simulink subsystem "FTireTiresFront"  (R2025b)
settings: Solver=VariableStepAuto  StartTime=0.0  StopTime=10.0  RelTol=1e-3
undefined symbols (not defined in the file): PlntWhlPrsFrnt, PlntWhlUnldRadiusFrnt
libraries: ftire_link x2, autolibsharedcoupling x1, autolibutils x1, vehdynlibtirecommon x1
settings Model: ModifiedByFormat=The MathWorks, Inc.  Creator=The MathWorks, Inc.  LastModifiedBy=The MathWorks, Inc.
settings OptimizationCC: ReuseModelBlockBuffer=off
settings RTWCC: GPUComputeCapability=3.5

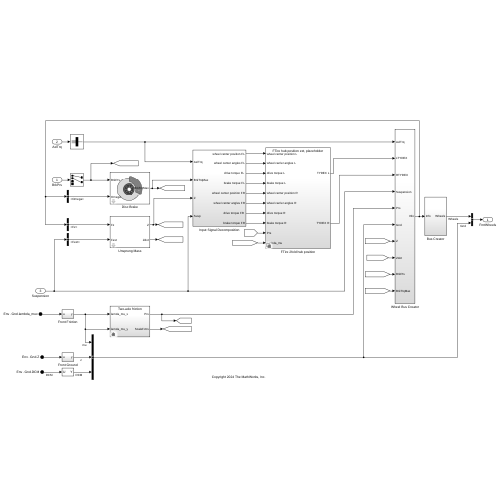
[thumbnail: Simulink's stored preview of the top-level diagram]
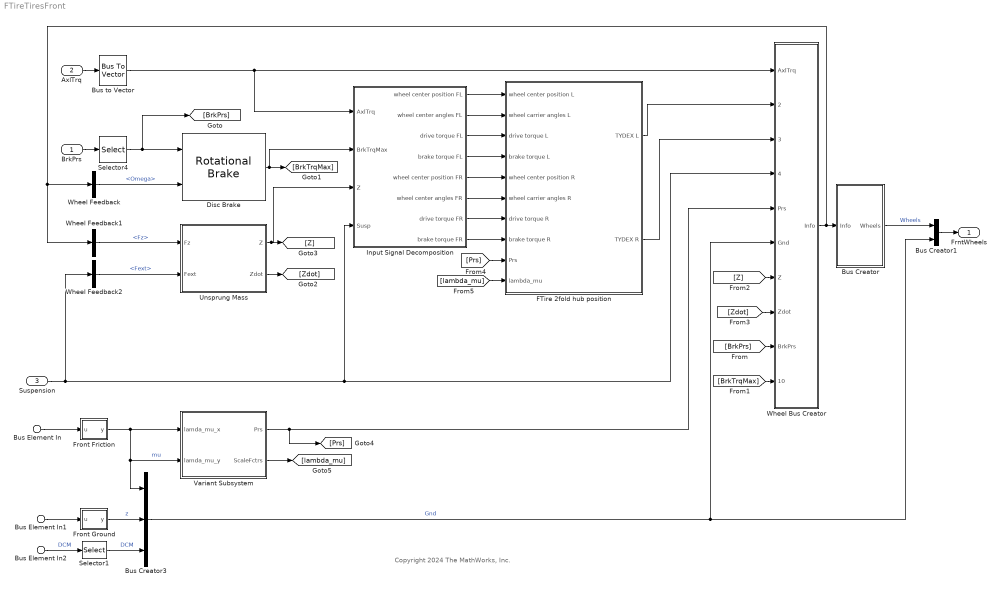
== system FTireTiresFront ==
  note: Copyright 2024 The MathWorks, Inc.
  BrkPrs : Inport
  AxlTrq : Inport  Port=2
  Suspension : Inport  Port=3
  Bus Element In : Inport  Port=4  PortName=Env  Element=Gnd.lambda_mux
  Bus Element In1 : Inport  Port=4  PortName=Env  Element=Gnd.Z
  Bus Element In2 : Inport  Port=4  PortName=Env  Element=Gnd.DCM
  Bus Creator1 : BusCreator  Inputs=2
  Bus Creator3 : BusCreator  Inputs=3
  Bus Creator : Subsystem
  Bus to Vector : BusToVector
  Disc Brake : autolibsharedcoupling/Rotational Brake  BrakeType=Disc  rotType=No inertia  extInfo=off  Iyy=1  br=1e-3  omegao=0  mu_static=PlntBrkStcFricCffFrnt  mu_kinetic=PlntBrkKinFricCffFrnt  disk_abore=PlntBrkActrBoreFrnt  Rm=PlntBrkPadMeanRadiusFrnt  num_pads=PlntBrkNumPadsFrnt  drum_abore=0.0508  drum_a=0.123  drum_c=0.212  drum_r=0.15  drum_theta1=0  drum_theta2=126  brake_p_bpt=[1 11.4736842105263 21.9473684210526 32.4210526315789 42.8947368421053 53.3684210526316 63.8421052631579 74.3157894736842 84.7894736842105 95.2631578947368 105.736842105263 116.210526315789 126.684210526316 137.157894736842 147.631578947368 158.105263157895 168.578947368421 179.052631578947 189.526315789474 200]  brake_n_bpt=[0 52.6315789473684 105.263157894737 157.894736842105 210.526315789474 263.157894736842 315.789473684211 368.421052631579 421.052631578947 473.684210526316 526.315789473684 578.947368421053 631.578947368421 684.210526315789 736.842105263158 789.473684210526 842.105263157895 894.736842105263 947.368421052632 1000]  f_brake_t=[43.4900602404453 42.5056030554862 41.5350898940194 40.5780454442085 39.6340111501808 38.7025443887544 37.7832176914519 36.8756180088306 35.9793460143796 35.0940154454303 34.2192524787115 33.3546951383474 32.4999927342521 31.6548053290159 30.8188032315107 29.991666515561 29.1730845621415 28.362755623661 27.5603864089927 26.765691687993;498.991217495636 487.695866636631 476.560505099801 465.579679307235 454.748127933653 444.060772460445 433.51270824929 423.099196101319 412.81565427025 402.657650900201 392.620896861006 382.701238955775 372.894653477208 363.197240090814 353.605216024701 344.114910546964 334.722759712992 325.425301366216 316.219170376863 307.10109410434;954.492374750826 932.886130217776 911.585920305583 890.581313170261 869.862244717126 849.419000532136 829.242198807128 809.322774193808 789.651962526121 770.221286354971 751.0225412433 732.047782773203 713.289314220164 694.739674852612 676.391628817892 658.238154578366 640.272434863842 622.48784710877 604.877954344734 587.436496520688;1409.99353200602 1378.07639379892 1346.61133551136 1315.58294703329 1284.9763615006 1254.77722860383 1224.97168936497 1195.5463522863 1166.48827078199 1137.78492180974 1109.42418562559 1081.39432659063 1053.68397496312 1026.28210961441 999.178041611083 972.361398609768 945.822110014692 919.550392851325 893.536738312604 867.771898937035;1865.49468926121 1823.26665738007 1781.63675071715 1740.58458089631 1700.09047828407 1660.13545667552 1620.7011799228 1581.76993037878 1543.32457903786 1505.34855726451 1467.82583000789 1430.74087040806 1394.07863570608 1357.82454437621 1321.96445440427 1286.48464264117 1251.37178516554 1216.61293859388 1182.19552228048 1148.10730135338;2320.9958465164 2268.45692096121 2216.66216592293 2165.58621475934 2115.20459506754 2065.49368474721 2016.43067048064 1967.99350847127 1920.16088729373 1872.91219271928 1826.22747439018 1780.08741422549 1734.47329644903 1689.36697913801 1644.75086719747 1600.60788667257 1556.92146031639 1513.67548433643 1470.85430624835 1428.44270376973;2776.49700377159 2713.64718454235 2651.68758112871 2590.58784862237 2530.31871185102 2470.8519128189 2412.16016103848 2354.21708656376 2296.9971955496 2240.47582817405 2184.62911877248 2129.43395804292 2074.86795719199 2020.9094138998 1967.53727999066 1914.73113070398 1862.47113546724 1810.73803007899 1759.51309021622 1708.77810618608;3231.99816102678 3158.8374481235 3086.71299633449 3015.58948248539 2945.43282863449 2876.21014089059 2807.88965159632 2740.44066465625 2673.83350380547 2608.03946362882 2543.03076315477 2478.78050186034 2415.26261793494 2352.4518486616 2290.32369278385 2228.85437473538 2168.02081061809 2107.80057582154 2048.17187418409 1989.11350860242;3687.49931828197 3604.02771170464 3521.73841154027 3440.59111634842 3360.54694541796 3281.56836896228 3203.61914215416 3126.66424274874 3050.66981206134 2975.60309908359 2901.43240753707 2828.12704567777 2755.6572786779 2683.9942834234 2613.11010557704 2542.97761876678 2473.57048576894 2404.8631215641 2336.83065815196 2269.44891101877;4143.00047553716 4049.21797528579 3956.76382674606 3865.59275021144 3775.66106220143 3686.92659703397 3599.34863271199 3512.88782084123 3427.50612031721 3343.16673453836 3259.83405191936 3177.4735894952 3096.05193942085 3015.5367181852 2935.89651837023 2857.10086279818 2779.12016091979 2701.92566730665 2625.48944211983 2549.78431343512;4598.50163279235 4494.40823886693 4391.78924195184 4290.59438407447 4190.77517898491 4092.28482510566 3995.07812326983 3899.11139893372 3804.34242857308 3710.73036999313 3618.23569630166 3526.82013331263 3436.44660016381 3347.079152947 3258.68293116342 3171.22410682959 3084.66983607064 2998.98821304921 2914.1482260877 2830.11971585147;5054.00279004754 4939.59850244808 4826.81465715762 4715.59601793749 4605.88929576838 4497.64305317735 4390.80761382767 4285.3349770262 4181.17873682896 4078.2940054479 3976.63734068395 3876.16667713006 3776.84126090677 3678.62158770879 3581.46934395661 3485.34735086099 ...(+2764 chars)]  aMode=2
  FTire 2fold hub position : Subsystem  Variant=on  VariantControlMode=label  VariantControl=Subsystem  LabelModeActiveChoice=FTire hub position ext, placeholder
  Front Friction : Subsystem
  Front Ground : Subsystem
  Input Signal Decomposition : Subsystem
  Selector1 : Selector  NumberOfDimensions=3  IndexOptions=Index vector (dialog),Index vector (dialog),Index vector (dialog)  Indices=[1 2 3],[1 2 3],[1 2]  OutputSizes=1,1,1
  Selector4 : Selector  InputPortWidth=4  IndexOptions=Index vector (dialog)  Indices=[1 2]  OutputSizes=1
  Unsprung Mass : Subsystem  mask{m=30, b=10e3}
      mask prompts: m "Unsprung mass, [kg]"; b "Unsprung damping [Ns/m]"
  Variant Subsystem : Subsystem  Variant=on  VariantControlMode=label  LabelModeActiveChoice=TwoAxleFriction
  Wheel Bus Creator : Subsystem
  Wheel Feedback : BusSelector  OutputSignals=Omega
  Wheel Feedback1 : BusSelector  OutputSignals=Fz
  Wheel Feedback2 : BusSelector  OutputSignals=Fext
  FrntWheels : Outport  VectorParamsAs1DForOutWhenUnconnected=off
  wires:
  [Z] -> Wheel Bus Creator/7(Z)
  Wheel Feedback2/1 -> Unsprung Mass/2(Fext)  "<Fext>"
  Wheel Bus Creator/1(Info) -> Wheel Feedback1/1, Wheel Feedback/1, Bus Creator/1(Info)
  [Zdot] -> Wheel Bus Creator/8(Zdot)
  Suspension/1 -> Wheel Feedback2/1, Input Signal Decomposition/4(Susp), Wheel Bus Creator/4(Suspension)
  Wheel Feedback1/1 -> Unsprung Mass/1(Fz)  "<Fz>"
  Unsprung Mass/1(Z) -> Input Signal Decomposition/3(Z), [Z]
  Unsprung Mass/2(Zdot) -> [Zdot]
  Bus Element In1/1 -> Front Ground/1(u)
  AxlTrq/1 -> Bus to Vector/1
  Bus Element In/1 -> Front Friction/1(u)
  Bus Creator3/1 -> Wheel Bus Creator/6(Gnd), Bus Creator1/2  "Gnd"
  Bus Creator1/1 -> FrntWheels/1
  Front Ground/1(y) -> Bus Creator3/2  "z"
  Front Friction/1(y) -> Variant Subsystem/2(lamda_mu_y), Bus Creator3/1, Variant Subsystem/1(lamda_mu_x)  "mu"
  BrkPrs/1 -> Selector4/1
  Wheel Feedback/1 -> Disc Brake/2  "<Omega>"
  Bus to Vector/1 -> Input Signal Decomposition/1(AxlTrq), Wheel Bus Creator/1(AxlTrq)
  Selector4/1 -> [BrkPrs], Disc Brake/1
  Bus Element In2/1 -> Selector1/1  "DCM"
  Selector1/1 -> Bus Creator3/3  "DCM"
  Bus Creator/1(Wheels) -> Bus Creator1/1  "Wheels"
  Input Signal Decomposition/1(wheel center position FL) -> FTire 2fold hub position/1(wheel center position L)
  Input Signal Decomposition/2(wheel center angles FL) -> FTire 2fold hub position/2(wheel carrier angles L)
  Input Signal Decomposition/3("drive torque FL ") -> FTire 2fold hub position/3(drive torque L)
  Input Signal Decomposition/4(brake torque FL) -> FTire 2fold hub position/4(brake torque L)
  Input Signal Decomposition/5(wheel center position FR) -> FTire 2fold hub position/5(wheel center position R)
  Input Signal Decomposition/6(wheel center angles FR) -> FTire 2fold hub position/6(wheel carrier angles R)
  Input Signal Decomposition/7("drive torque FR ") -> FTire 2fold hub position/7(drive torque R)
  Input Signal Decomposition/8(brake torque FR) -> FTire 2fold hub position/8(brake torque R)
  FTire 2fold hub position/1(TYDEX L) -> Wheel Bus Creator/2(LTYDEX)
  FTire 2fold hub position/2(TYDEX R) -> Wheel Bus Creator/3(RTYDEX)
  Variant Subsystem/2(ScaleFctrs) -> [lambda_mu]
  [BrkPrs] -> Wheel Bus Creator/9(BrkPrs)
  [BrkTrqMax] -> Wheel Bus Creator/10(BrkTrqMax)
  Disc Brake/1 -> [BrkTrqMax], Input Signal Decomposition/2(BrkTrqMax)
  [Prs] -> FTire 2fold hub position/9(Prs)
  Variant Subsystem/1(Prs) -> [Prs], Wheel Bus Creator/5(Prs)
  [lambda_mu] -> FTire 2fold hub position/10(lambda_mu)

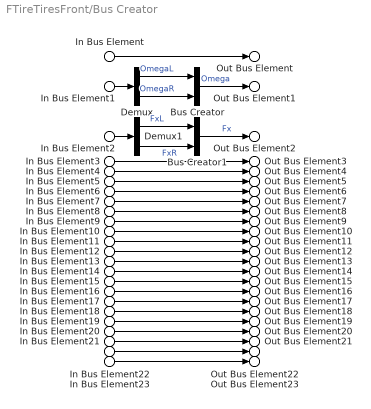
== system FTireTiresFront/Bus Creator ==
  In Bus Element : Inport  PortName=Info  Element=AxlTrq
  In Bus Element1 : Inport  PortName=Info  Element=Omega
  In Bus Element2 : Inport  PortName=Info  Element=Fx
  In Bus Element3 : Inport  PortName=Info  Element=Fy
  In Bus Element4 : Inport  PortName=Info  Element=Fz
  In Bus Element5 : Inport  PortName=Info  Element=Mx
  In Bus Element6 : Inport  PortName=Info  Element=My
  In Bus Element7 : Inport  PortName=Info  Element=Mz
  In Bus Element8 : Inport  PortName=Info  Element=Vx
  In Bus Element9 : Inport  PortName=Info  Element=Vy
  In Bus Element10 : Inport  PortName=Info  Element=Re
  In Bus Element11 : Inport  PortName=Info  Element=Kappa
  In Bus Element12 : Inport  PortName=Info  Element=Alpha
  In Bus Element13 : Inport  PortName=Info  Element=a
  In Bus Element14 : Inport  PortName=Info  Element=b
  In Bus Element15 : Inport  PortName=Info  Element=Gamma
  In Bus Element16 : Inport  PortName=Info  Element=psidot
  In Bus Element17 : Inport  PortName=Info  Element=BrkTrq
  In Bus Element18 : Inport  PortName=Info  Element=BrkPrs
  In Bus Element19 : Inport  PortName=Info  Element=z
  In Bus Element20 : Inport  PortName=Info  Element=zdot
  In Bus Element21 : Inport  PortName=Info  Element=Gnd
  In Bus Element22 : Inport  PortName=Info  Element=GndFz
  In Bus Element23 : Inport  PortName=Info  Element=Prs
  Bus Creator : BusCreator  Inputs=2
  Bus Creator1 : BusCreator  Inputs=2
  Demux : Demux  Outputs=2
  Demux1 : Demux  Outputs=2
  Out Bus Element : Outport  PortName=Wheels  Element=AxlTrq
  Out Bus Element1 : Outport  PortName=Wheels  Element=Omega
  Out Bus Element2 : Outport  PortName=Wheels  Element=Fx
  Out Bus Element3 : Outport  PortName=Wheels  Element=Fy
  Out Bus Element4 : Outport  PortName=Wheels  Element=Fz
  Out Bus Element5 : Outport  PortName=Wheels  Element=Mx
  Out Bus Element6 : Outport  PortName=Wheels  Element=My
  Out Bus Element7 : Outport  PortName=Wheels  Element=Mz
  Out Bus Element8 : Outport  PortName=Wheels  Element=Vx
  Out Bus Element9 : Outport  PortName=Wheels  Element=Vy
  Out Bus Element10 : Outport  PortName=Wheels  Element=Re
  Out Bus Element11 : Outport  PortName=Wheels  Element=Kappa
  Out Bus Element12 : Outport  PortName=Wheels  Element=Alpha
  Out Bus Element13 : Outport  PortName=Wheels  Element=a
  Out Bus Element14 : Outport  PortName=Wheels  Element=b
  Out Bus Element15 : Outport  PortName=Wheels  Element=Gamma
  Out Bus Element16 : Outport  PortName=Wheels  Element=psidot
  Out Bus Element17 : Outport  PortName=Wheels  Element=BrkTrq
  Out Bus Element18 : Outport  PortName=Wheels  Element=BrkPrs
  Out Bus Element19 : Outport  PortName=Wheels  Element=z
  Out Bus Element20 : Outport  PortName=Wheels  Element=zdot
  Out Bus Element21 : Outport  PortName=Wheels  Element=Gnd
  Out Bus Element22 : Outport  PortName=Wheels  Element=GndFz
  Out Bus Element23 : Outport  PortName=Wheels  Element=Prs
  wires:
  In Bus Element16/1 -> Out Bus Element16/1
  In Bus Element10/1 -> Out Bus Element10/1
  In Bus Element3/1 -> Out Bus Element3/1
  In Bus Element18/1 -> Out Bus Element18/1
  In Bus Element12/1 -> Out Bus Element12/1
  In Bus Element11/1 -> Out Bus Element11/1
  In Bus Element20/1 -> Out Bus Element20/1
  In Bus Element13/1 -> Out Bus Element13/1
  In Bus Element8/1 -> Out Bus Element8/1
  In Bus Element14/1 -> Out Bus Element14/1
  In Bus Element15/1 -> Out Bus Element15/1
  In Bus Element17/1 -> Out Bus Element17/1
  In Bus Element19/1 -> Out Bus Element19/1
  In Bus Element22/1 -> Out Bus Element22/1
  In Bus Element21/1 -> Out Bus Element21/1
  In Bus Element23/1 -> Out Bus Element23/1
  In Bus Element1/1 -> Demux/1
  In Bus Element/1 -> Out Bus Element/1
  In Bus Element4/1 -> Out Bus Element4/1
  In Bus Element6/1 -> Out Bus Element6/1
  In Bus Element5/1 -> Out Bus Element5/1
  In Bus Element9/1 -> Out Bus Element9/1
  In Bus Element7/1 -> Out Bus Element7/1
  Demux/1 -> Bus Creator/1  "OmegaL"
  Demux/2 -> Bus Creator/2  "OmegaR"
  Bus Creator/1 -> Out Bus Element1/1  "Omega"
  Bus Creator1/1 -> Out Bus Element2/1  "Fx"
  Demux1/2 -> Bus Creator1/2  "FxR"
  Demux1/1 -> Bus Creator1/1  "FxL"
  In Bus Element2/1 -> Demux1/1

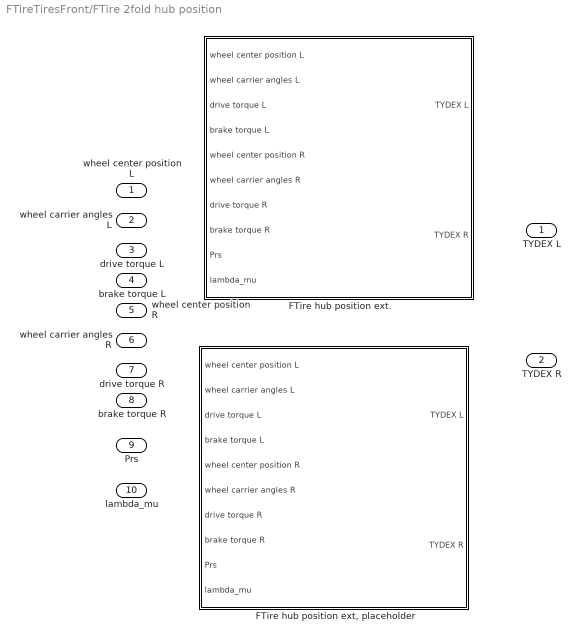
== system FTireTiresFront/FTire 2fold hub position ==
  wheel center position L : Inport
  wheel carrier angles L : Inport  Port=2
  drive torque L : Inport  Port=3
  brake torque L : Inport  Port=4
  wheel center position R : Inport  Port=5
  wheel carrier angles R : Inport  Port=6
  drive torque R : Inport  Port=7
  brake torque R : Inport  Port=8
  Prs : Inport  Port=9
  lambda_mu : Inport  Port=10
  "FTire hub position ext, placeholder" : Subsystem  VariantControl=FTire hub position ext, placeholder
  FTire hub position ext. : Subsystem  VariantControl=FTire hub position ext.
  TYDEX L : Outport
  TYDEX R : Outport  Port=2

== system FTireTiresFront/Front Friction ==
  u : Inport
  Selector1 : Selector  InputPortWidth=4  IndexOptions=Index vector (dialog)  Indices=[1 2]  OutputSizes=1
  y : Outport
  wires:
  u/1 -> Selector1/1
  Selector1/1 -> y/1

== system FTireTiresFront/Front Ground ==
  u : Inport
  Selector1 : Selector  InputPortWidth=4  IndexOptions=Index vector (dialog)  Indices=[1 2]  OutputSizes=1
  y : Outport
  wires:
  Selector1/1 -> y/1
  u/1 -> Selector1/1

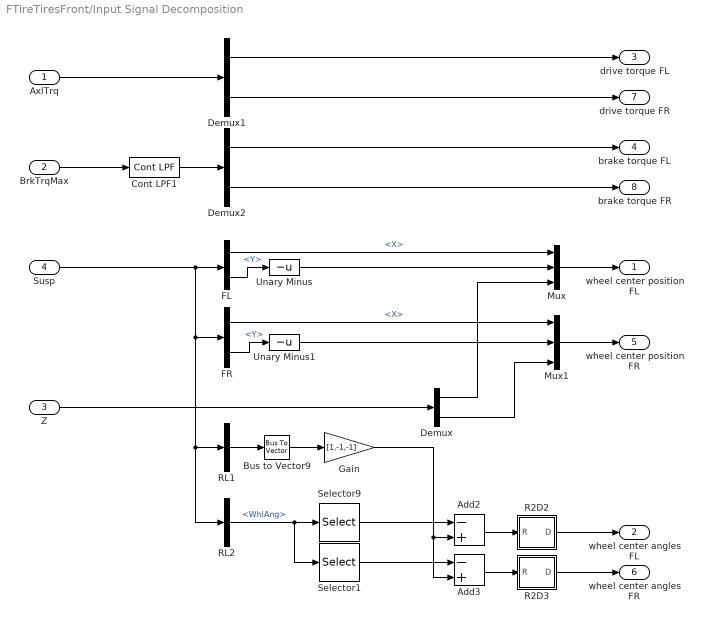
== system FTireTiresFront/Input Signal Decomposition ==
  AxlTrq : Inport
  BrkTrqMax : Inport  Port=2
  Z : Inport  Port=3
  Susp : Inport  Port=4
  Add2 : Sum  Inputs=-+
  Add3 : Sum  Inputs=-+
  Bus to Vector9 : BusToVector
  Cont LPF1 : autolibutils/Cont LPF  wc=100*2*pi  AbsoluteTolerance=auto  aMode=2
  Demux : Demux  Outputs=2
  Demux1 : Demux  Outputs=2
  Demux2 : Demux  Outputs=2
  FL : BusSelector  OutputSignals=Veh.InertFrm.FrntAxl.Lft.Disp.X,Veh.InertFrm.FrntAxl.Lft.Disp.Y
  FR : BusSelector  OutputSignals=Veh.InertFrm.FrntAxl.Rght.Disp.X,Veh.InertFrm.FrntAxl.Rght.Disp.Y
  Gain : Gain  Gain=[1,-1,-1]
  Mux : Mux  Inputs=3
  Mux1 : Mux  Inputs=3
  R2D2 : Subsystem
  R2D3 : Subsystem
  RL1 : BusSelector  OutputSignals=Veh.InertFrm.Cg.Ang.phi,Veh.InertFrm.Cg.Ang.theta,Veh.InertFrm.Cg.Ang.psi  OutputAsBus=on
  RL2 : BusSelector  OutputSignals=WhlAng
  Selector1 : Selector  NumberOfDimensions=2  InputPortWidth=4  IndexOptions=Index vector (dialog),Index vector (dialog)  Indices=[1 2 3],[2]  OutputSizes=1,1
  Selector9 : Selector  NumberOfDimensions=2  InputPortWidth=4  IndexOptions=Index vector (dialog),Index vector (dialog)  Indices=[1 2 3],[1]  OutputSizes=1,1
  Unary Minus : UnaryMinus
  Unary Minus1 : UnaryMinus
  wheel center position FL : Outport
  wheel center angles FL : Outport  Port=2
  "drive torque FL " : Outport  Port=3
  brake torque FL : Outport  Port=4
  wheel center position FR : Outport  Port=5
  wheel center angles FR : Outport  Port=6
  "drive torque FR " : Outport  Port=7
  brake torque FR : Outport  Port=8
  wires:
  Cont LPF1/1 -> Demux2/1
  Demux/1 -> Mux/3
  Demux/2 -> Mux1/3
  Susp/1 -> RL2/1, RL1/1, FR/1, FL/1
  FL/2 -> Unary Minus/1  "<Y>"
  Unary Minus1/1 -> Mux1/2
  Mux1/1 -> wheel center position FR/1
  Unary Minus/1 -> Mux/2
  FL/1 -> Mux/1  "<X>"
  FR/1 -> Mux1/1  "<X>"
  Demux1/2 -> "drive torque FR "/1
  Demux1/1 -> "drive torque FL "/1
  AxlTrq/1 -> Demux1/1
  Mux/1 -> wheel center position FL/1
  Demux2/2 -> brake torque FR/1
  Demux2/1 -> brake torque FL/1
  BrkTrqMax/1 -> Cont LPF1/1
  Gain/1 -> Add3/2, Add2/2
  Selector1/1 -> Add3/1
  RL2/1 -> Selector9/1, Selector1/1  "<WhlAng>"
  Add3/1 -> R2D3/1(R)
  RL1/1 -> Bus to Vector9/1
  Selector9/1 -> Add2/1
  Add2/1 -> R2D2/1(R)
  Bus to Vector9/1 -> Gain/1
  R2D2/1(D) -> wheel center angles FL/1
  R2D3/1(D) -> wheel center angles FR/1
  FR/2 -> Unary Minus1/1  "<Y>"
  Z/1 -> Demux/1

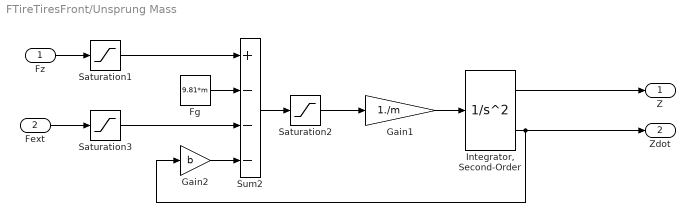
== system FTireTiresFront/Unsprung Mass ==
  Fz : Inport
  Fext : Inport  Port=2
  Fg : Constant  Value=9.81*m
  Gain1 : Gain  Gain=1./m  SaturateOnIntegerOverflow=on  OutDataTypeStr=Inherit: Same as input  ParamDataTypeStr=Inherit: Same as input
  Gain2 : Gain  Gain=b  SaturateOnIntegerOverflow=on  OutDataTypeStr=Inherit: Same as input  ParamDataTypeStr=Inherit: Same as input
  "Integrator, Second-Order" : SecondOrderIntegrator  ICX=ones(2,1).*0.00  LimitX=on  UpperLimitX=0.02  LowerLimitX=-.02  ICDXDT=0
  Saturation1 : Saturate  UpperLimit=10e3  LowerLimit=0  ZeroCross=off
  Saturation2 : Saturate  UpperLimit=100  LowerLimit=-100  ZeroCross=off
  Saturation3 : Saturate  UpperLimit=10e3  LowerLimit=0  ZeroCross=off
  Sum2 : Sum  Inputs=+---  InputSameDT=on  SaturateOnIntegerOverflow=on  OutDataTypeStr=Inherit: Same as first input
  Z : Outport
  Zdot : Outport  Port=2
  wires:
  "Integrator, Second-Order"/1 -> Z/1
  Fext/1 -> Saturation3/1
  Saturation2/1 -> Gain1/1
  Sum2/1 -> Saturation2/1
  Gain1/1 -> "Integrator, Second-Order"/1
  Saturation3/1 -> Sum2/3
  "Integrator, Second-Order"/2 -> Gain2/1, Zdot/1
  Gain2/1 -> Sum2/4
  Fz/1 -> Saturation1/1
  Fg/1 -> Sum2/2
  Saturation1/1 -> Sum2/1

== system FTireTiresFront/Variant Subsystem ==
  note: 1) Add Subsystem or Model blocks as valid variant choices.
      | 2) You cannot connect blocks at this level. At simulation, connectivity is automatically
      | determined, based on the active variant and port name matching.
  lamda_mu_x : Inport
  lamda_mu_y : Inport  Port=2
  Two-axle friction : Subsystem  VariantControl=TwoAxleFriction
  Prs : Outport
  ScaleFctrs : Outport  Port=2

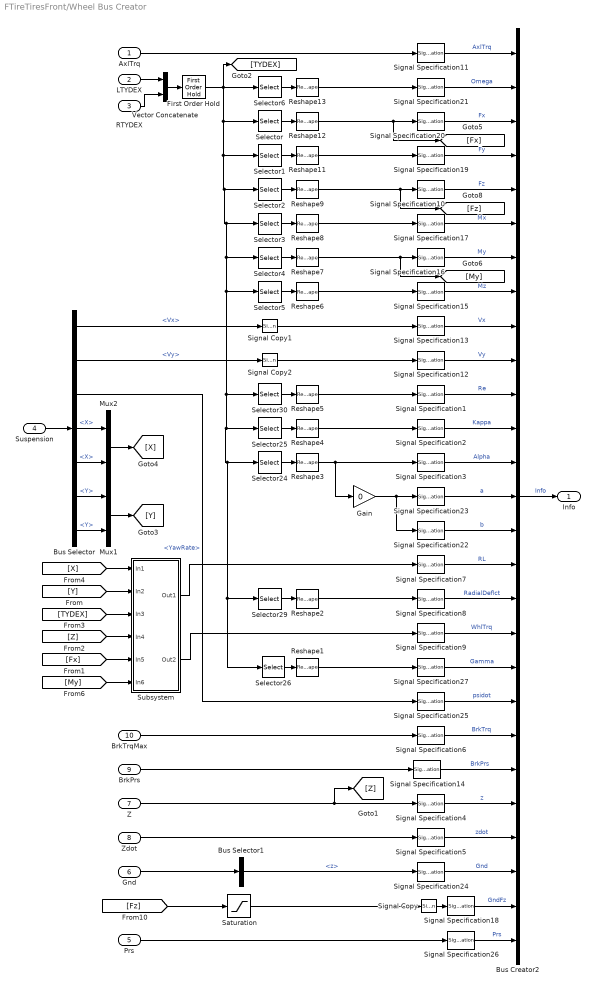
== system FTireTiresFront/Wheel Bus Creator ==
  AxlTrq : Inport
  LTYDEX : Inport  Port=2
  RTYDEX : Inport  Port=3
  Suspension : Inport  Port=4
  Prs : Inport  Port=5
  Gnd : Inport  Port=6
  Z : Inport  Port=7
  Zdot : Inport  Port=8
  BrkPrs : Inport  Port=9
  BrkTrqMax : Inport  Port=10
  Bus Creator2 : BusCreator  Inputs=27
  Bus Selector : BusSelector  OutputSignals=Vx,Vy,YawRate,Veh.InertFrm.FrntAxl.Lft.Disp.X,Veh.InertFrm.FrntAxl.Rght.Disp.X,Veh.InertFrm.RearAxl.Lft.Disp.Y,Veh.InertFrm.RearAxl.Rght.Disp.Y
  Bus Selector1 : BusSelector  OutputSignals=z
  First Order Hold : FirstOrderHold  ErrorTolerance=inf
  Gain : Gain  Gain=0
  Mux1 : Mux  Inputs=2
  Mux2 : Mux  Inputs=2
  Reshape{1..9,11..13} (12 alike) : Reshape
  Saturation : Saturate  UpperLimit=inf  LowerLimit=0  ZeroCross=off
  Selector : Selector  NumberOfDimensions=2  IndexOptions=Index vector (dialog),Select all  Indices=[1],1  OutputSizes=1,1
  Selector1 : Selector  NumberOfDimensions=2  IndexOptions=Index vector (dialog),Select all  Indices=[2],1  OutputSizes=1,1
  Selector2 : Selector  NumberOfDimensions=2  IndexOptions=Index vector (dialog),Select all  Indices=[3],1  OutputSizes=1,1
  Selector24 : Selector  NumberOfDimensions=2  IndexOptions=Index vector (dialog),Select all  Indices=7,1  OutputSizes=1,1
  Selector25 : Selector  NumberOfDimensions=2  IndexOptions=Index vector (dialog),Select all  Indices=8,1  OutputSizes=1,1
  Selector26 : Selector  NumberOfDimensions=2  IndexOptions=Index vector (dialog),Select all  Indices=9,1  OutputSizes=1,1
  Selector29 : Selector  NumberOfDimensions=2  IndexOptions=Index vector (dialog),Select all  Indices=44,1  OutputSizes=1,1
  Selector3 : Selector  NumberOfDimensions=2  IndexOptions=Index vector (dialog),Select all  Indices=[4],1  OutputSizes=1,1
  Selector30 : Selector  NumberOfDimensions=2  IndexOptions=Index vector (dialog),Select all  Indices=90,1  OutputSizes=1,1
  Selector4 : Selector  NumberOfDimensions=2  IndexOptions=Index vector (dialog),Select all  Indices=[5],1  OutputSizes=1,1
  Selector5 : Selector  NumberOfDimensions=2  IndexOptions=Index vector (dialog),Select all  Indices=[6],1  OutputSizes=1,1
  Selector6 : Selector  NumberOfDimensions=2  IndexOptions=Index vector (dialog),Select all  Indices=[50],1  OutputSizes=1,1
  Signal Copy : SignalConversion  OverrideOpt=off
  Signal Copy1 : SignalConversion  OverrideOpt=off
  Signal Copy2 : SignalConversion  OverrideOpt=off
  Signal Specification{1,4,7..8,22..24} (7 alike) : SignalSpecification  Unit=m
  Signal Specification{10,18..20} (4 alike) : SignalSpecification  Unit=N
  Signal Specification{6,9,11,15..17} (6 alike) : SignalSpecification  Unit=N*m
  Signal Specification12 : SignalSpecification  Unit=m/s
  Signal Specification13 : SignalSpecification  Unit=m/s
  Signal Specification14 : SignalSpecification  Unit=Pa
  Signal Specification2 : SignalSpecification  Unit=1
  Signal Specification21 : SignalSpecification  Unit=rad/s
  Signal Specification25 : SignalSpecification  Unit=rad/s
  Signal Specification26 : SignalSpecification  Unit=Pa
  Signal Specification27 : SignalSpecification  Unit=rad
  Signal Specification3 : SignalSpecification  Unit=rad
  Signal Specification5 : SignalSpecification  Unit=m/s
  Subsystem : Subsystem
  Vector Concatenate : Concatenate  Mode=Multidimensional array  ConcatenateDimension=2
  Info : Outport
  wires:
  First Order Hold/1 -> Selector/1, Selector1/1, Selector2/1, Selector3/1, Selector4/1, Selector5/1, Selector26/1, Selector29/1, Selector24/1, Selector25/1, Selector30/1, [TYDEX], Selector6/1
  Z/1 -> [Z], Signal Specification4/1
  Saturation/1 -> Signal Copy/1
  Reshape13/1 -> Signal Specification21/1
  Reshape12/1 -> [Fx], Signal Specification20/1
  Reshape9/1 -> Signal Specification10/1, [Fz]
  Reshape11/1 -> Signal Specification19/1
  Reshape8/1 -> Signal Specification17/1
  Reshape7/1 -> [My], Signal Specification16/1
  Reshape6/1 -> Signal Specification15/1
  Reshape5/1 -> Signal Specification1/1
  Reshape4/1 -> Signal Specification2/1
  Reshape3/1 -> Gain/1, Signal Specification3/1
  Reshape1/1 -> Signal Specification27/1
  Reshape2/1 -> Signal Specification8/1
  Prs/1 -> Signal Specification26/1
  Mux2/1 -> [X]
  Bus Selector/5 -> Mux2/2  "<X>"
  Bus Selector/4 -> Mux2/1  "<X>"
  Bus Selector/6 -> Mux1/1  "<Y>"
  Bus Selector/7 -> Mux1/2  "<Y>"
  Mux1/1 -> [Y]
  Suspension/1 -> Bus Selector/1
  Bus Selector/1 -> Signal Copy1/1  "<Vx>"
  Bus Selector/2 -> Signal Copy2/1  "<Vy>"
  Selector6/1 -> Reshape13/1
  Selector/1 -> Reshape12/1
  Selector1/1 -> Reshape11/1
  Selector2/1 -> Reshape9/1
  Selector3/1 -> Reshape8/1
  Selector4/1 -> Reshape7/1
  Selector5/1 -> Reshape6/1
  Signal Specification15/1 -> Bus Creator2/8  "Mz"
  Signal Specification20/1 -> Bus Creator2/3  "Fx"
  Signal Specification4/1 -> Bus Creator2/23  "z"
  Signal Specification9/1 -> Bus Creator2/18  "WhlTrq"
  Signal Specification19/1 -> Bus Creator2/4  "Fy"
  Signal Specification3/1 -> Bus Creator2/13  "Alpha"
  Signal Specification23/1 -> Bus Creator2/14  "a"
  RTYDEX/1 -> Vector Concatenate/2
  Signal Specification6/1 -> Bus Creator2/21  "BrkTrq"
  Signal Specification22/1 -> Bus Creator2/15  "b"
  Signal Specification2/1 -> Bus Creator2/12  "Kappa"
  Signal Specification18/1 -> Bus Creator2/26  "GndFz"
  Signal Specification11/1 -> Bus Creator2/1  "AxlTrq"
  Signal Specification5/1 -> Bus Creator2/24  "zdot"
  Signal Copy/1 -> Signal Specification18/1
  Signal Specification7/1 -> Bus Creator2/16  "RL"
  Bus Creator2/1 -> Info/1  "Info"
  Signal Specification1/1 -> Bus Creator2/11  "Re"
  Signal Specification16/1 -> Bus Creator2/7  "My"
  Signal Specification10/1 -> Bus Creator2/5  "Fz"
  Signal Specification17/1 -> Bus Creator2/6  "Mx"
  Signal Specification21/1 -> Bus Creator2/2  "Omega"
  LTYDEX/1 -> Vector Concatenate/1
  Signal Specification8/1 -> Bus Creator2/17  "RadialDeflct"
  Gain/1 -> Signal Specification22/1, Signal Specification23/1
  AxlTrq/1 -> Signal Specification11/1
  Signal Specification26/1 -> Bus Creator2/27  "Prs"
  Signal Specification12/1 -> Bus Creator2/10  "Vy"
  Signal Specification24/1 -> Bus Creator2/25  "Gnd"
  Signal Specification13/1 -> Bus Creator2/9  "Vx"
  Signal Specification14/1 -> Bus Creator2/22  "BrkPrs"
  Signal Specification25/1 -> Bus Creator2/20  "psidot"
  Signal Copy2/1 -> Signal Specification12/1
  Signal Copy1/1 -> Signal Specification13/1
  Selector25/1 -> Reshape4/1
  Selector30/1 -> Reshape5/1
  Selector26/1 -> Reshape1/1
  Signal Specification27/1 -> Bus Creator2/19  "Gamma"
  Selector24/1 -> Reshape3/1
  Vector Concatenate/1 -> First Order Hold/1
  Selector29/1 -> Reshape2/1
  BrkPrs/1 -> Signal Specification14/1
  Gnd/1 -> Bus Selector1/1
  Bus Selector/3 -> Signal Specification25/1  "<YawRate>"
  Bus Selector1/1 -> Signal Specification24/1  "<z>"
  BrkTrqMax/1 -> Signal Specification6/1
  [X] -> Subsystem/1(In1)
  [Y] -> Subsystem/2(In2)
  [TYDEX] -> Subsystem/3(In3)
  [Z] -> Subsystem/4(In4)
  [Fx] -> Subsystem/5(In5)
  [My] -> Subsystem/6(In6)
  Subsystem/1(Out1) -> Signal Specification7/1
  Subsystem/2(Out2) -> Signal Specification9/1
  [Fz] -> Saturation/1
  Zdot/1 -> Signal Specification5/1

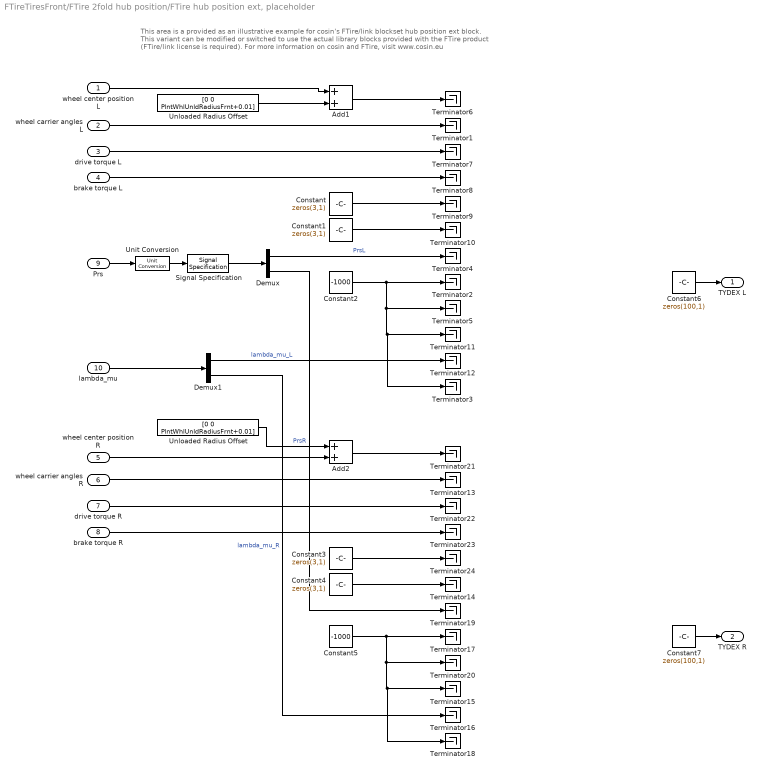
== system FTireTiresFront/FTire 2fold hub position/FTire hub position ext, placeholder ==
  note: This area is a provided as an illustrative example for cosin's FTire/link blockset hub position ext block.
      | This variant can be modified or switched to use the actual library blocks provided with the FTire product (FTire/link license is required).
      | For more information on cosin and FTire, visit www.cosin.eu
  wheel center position L : Inport
  wheel carrier angles L : Inport  Port=2
  drive torque L : Inport  Port=3
  brake torque L : Inport  Port=4
  wheel center position R : Inport  Port=5
  wheel carrier angles R : Inport  Port=6
  drive torque R : Inport  Port=7
  brake torque R : Inport  Port=8
  Prs : Inport  Port=9
  lambda_mu : Inport  Port=10
  Add1 : Sum
  Add2 : Sum
  Constant{,1,3..4} (4 alike) : Constant  Value=zeros(3,1)
  Constant2 : Constant  Value=-1000
  Constant5 : Constant  Value=-1000
  Constant6 : Constant  Value=zeros(100,1)
  Constant7 : Constant  Value=zeros(100,1)
  Demux : Demux  Outputs=2
  Demux1 : Demux  Outputs=2
  Signal Specification : SignalSpecification  Unit=bar
  Terminator{1..24} (24 alike) : Terminator
  Unit Conversion : UnitConversion
  Unloaded Radius Offset : Constant  Value=[0 0 PlntWhlUnldRadiusFrnt+0.01]
  "Unloaded Radius Offset " : Constant  Value=[0 0 PlntWhlUnldRadiusFrnt+0.01]
  TYDEX L : Outport
  TYDEX R : Outport  Port=2
  wires:
  Constant7/1 -> TYDEX R/1
  brake torque L/1 -> Terminator8/1
  Constant/1 -> Terminator9/1
  Constant1/1 -> Terminator10/1
  wheel center position R/1 -> Add2/2
  wheel carrier angles R/1 -> Terminator13/1
  drive torque R/1 -> Terminator22/1
  brake torque R/1 -> Terminator23/1
  Constant3/1 -> Terminator24/1
  Constant4/1 -> Terminator14/1
  Constant5/1 -> Terminator17/1, Terminator20/1, Terminator15/1, Terminator18/1
  Constant2/1 -> Terminator2/1, Terminator5/1, Terminator3/1, Terminator11/1
  wheel center position L/1 -> Add1/1
  drive torque L/1 -> Terminator7/1
  Add1/1 -> Terminator6/1
  wheel carrier angles L/1 -> Terminator1/1
  Constant6/1 -> TYDEX L/1
  Prs/1 -> Unit Conversion/1
  Signal Specification/1 -> Demux/1
  Demux/1 -> Terminator4/1  "PrsL"
  Demux/2 -> Terminator19/1  "PrsR"
  Demux1/2 -> Terminator16/1  "lambda_mu_R"
  Demux1/1 -> Terminator12/1  "lambda_mu_L"
  lambda_mu/1 -> Demux1/1
  Unloaded Radius Offset/1 -> Add1/2
  Add2/1 -> Terminator21/1
  "Unloaded Radius Offset "/1 -> Add2/1
  Unit Conversion/1 -> Signal Specification/1

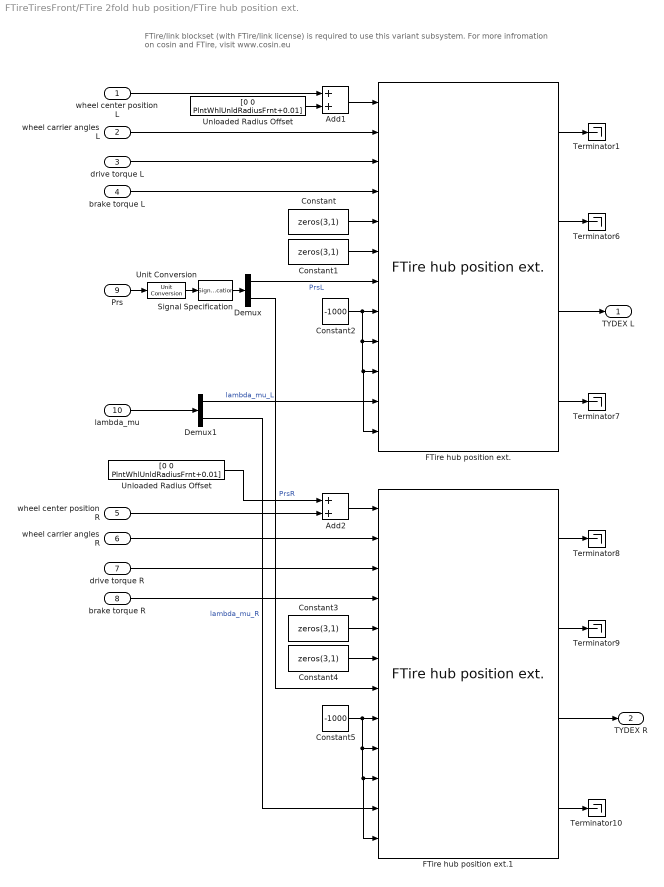
== system FTireTiresFront/FTire 2fold hub position/FTire hub position ext. ==
  note: FTire/link blockset (with FTire/link license) is required to use this variant subsystem.
      | For more infromation on cosin and FTire, visit www.cosin.eu
  wheel center position L : Inport
  wheel carrier angles L : Inport  Port=2
  drive torque L : Inport  Port=3
  brake torque L : Inport  Port=4
  wheel center position R : Inport  Port=5
  wheel carrier angles R : Inport  Port=6
  drive torque R : Inport  Port=7
  brake torque R : Inport  Port=8
  Prs : Inport  Port=9
  lambda_mu : Inport  Port=10
  Add1 : Sum
  Add2 : Sum
  Constant{,1,3..4} (4 alike) : Constant  Value=zeros(3,1)
  Constant2 : Constant  Value=-1000
  Constant5 : Constant  Value=-1000
  Demux : Demux  Outputs=2
  Demux1 : Demux  Outputs=2
  FTire hub position ext. : ftire_link/Extended Interface/FTire hub position ext.  fileti=C:\Program Files (x86)\cosin\2024-3\ftire\param\pass_car_245_45R19_98W.tir  filero=C:\Program Files (x86)\cosin\2024-3\roads\_default.rdf  fileplo=ftire.plo  mode=on  side=off  h=1  msg=on  anim=on  v0=[0 0 0]  w0=[0 0 0]
      settings: SourceProductName=FTire/link Blockset
  FTire hub position ext.1 : ftire_link/Extended Interface/FTire hub position ext.  fileti=C:\Program Files (x86)\cosin\2024-3\ftire\param\pass_car_245_45R19_98W.tir  filero=C:\Program Files (x86)\cosin\2024-3\roads\_default.rdf  fileplo=ftire.plo  mode=on  side=on  h=1  msg=on  anim=on  v0=[0 0 0]  w0=[0 0 0]
      settings: SourceProductName=FTire/link Blockset
  Signal Specification : SignalSpecification  Unit=bar
  Terminator{1,6..10} (6 alike) : Terminator
  Unit Conversion : UnitConversion
  Unloaded Radius Offset : Constant  Value=[0 0 PlntWhlUnldRadiusFrnt+0.01]
  "Unloaded Radius Offset " : Constant  Value=[0 0 PlntWhlUnldRadiusFrnt+0.01]
  TYDEX L : Outport
  TYDEX R : Outport  Port=2
  wires:
  FTire hub position ext./3 -> TYDEX L/1
  FTire hub position ext./1 -> Terminator1/1
  FTire hub position ext./2 -> Terminator6/1
  FTire hub position ext./4 -> Terminator7/1
  wheel center position L/1 -> Add1/1
  wheel carrier angles L/1 -> FTire hub position ext./2
  drive torque L/1 -> FTire hub position ext./3
  brake torque L/1 -> FTire hub position ext./4
  Constant/1 -> FTire hub position ext./5
  Constant1/1 -> FTire hub position ext./6
  Constant2/1 -> FTire hub position ext./12, FTire hub position ext./10, FTire hub position ext./9, FTire hub position ext./8
  Constant5/1 -> FTire hub position ext.1/8, FTire hub position ext.1/9, FTire hub position ext.1/10, FTire hub position ext.1/12
  brake torque R/1 -> FTire hub position ext.1/4
  drive torque R/1 -> FTire hub position ext.1/3
  wheel carrier angles R/1 -> FTire hub position ext.1/2
  wheel center position R/1 -> Add2/2
  FTire hub position ext.1/4 -> Terminator10/1
  FTire hub position ext.1/2 -> Terminator9/1
  FTire hub position ext.1/1 -> Terminator8/1
  FTire hub position ext.1/3 -> TYDEX R/1
  lambda_mu/1 -> Demux1/1
  Demux/1 -> FTire hub position ext./7  "PrsL"
  Demux1/1 -> FTire hub position ext./11  "lambda_mu_L"
  Prs/1 -> Unit Conversion/1
  Signal Specification/1 -> Demux/1
  Demux1/2 -> FTire hub position ext.1/11  "lambda_mu_R"
  Demux/2 -> FTire hub position ext.1/7  "PrsR"
  Constant3/1 -> FTire hub position ext.1/5
  Constant4/1 -> FTire hub position ext.1/6
  Add1/1 -> FTire hub position ext./1
  Unloaded Radius Offset/1 -> Add1/2
  Add2/1 -> FTire hub position ext.1/1
  "Unloaded Radius Offset "/1 -> Add2/1
  Unit Conversion/1 -> Signal Specification/1

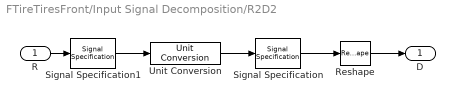
== system FTireTiresFront/Input Signal Decomposition/R2D2 ==
  R : Inport
  Reshape : Reshape
  Signal Specification : SignalSpecification  Unit=deg
  Signal Specification1 : SignalSpecification  Unit=rad
  Unit Conversion : UnitConversion
  D : Outport
  wires:
  Signal Specification1/1 -> Unit Conversion/1
  Unit Conversion/1 -> Signal Specification/1
  R/1 -> Signal Specification1/1
  Signal Specification/1 -> Reshape/1
  Reshape/1 -> D/1

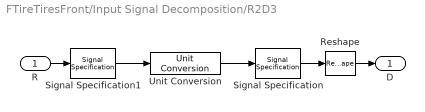
== system FTireTiresFront/Input Signal Decomposition/R2D3 ==
  R : Inport
  Reshape : Reshape
  Signal Specification : SignalSpecification  Unit=deg
  Signal Specification1 : SignalSpecification  Unit=rad
  Unit Conversion : UnitConversion
  D : Outport
  wires:
  Signal Specification/1 -> Reshape/1
  R/1 -> Signal Specification1/1
  Unit Conversion/1 -> Signal Specification/1
  Signal Specification1/1 -> Unit Conversion/1
  Reshape/1 -> D/1

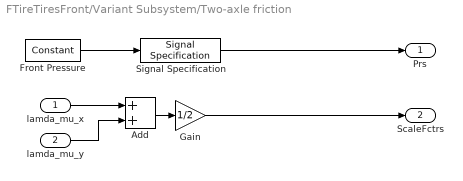
== system FTireTiresFront/Variant Subsystem/Two-axle friction ==
  lamda_mu_x : Inport
  lamda_mu_y : Inport  Port=2
  Add : Sum
  Front Pressure : vehdynlibtirecommon/Constant  const=PlntWhlPrsFrnt  numWheels=PlntWhlNumFrnt
  Gain : Gain  Gain=1/2
  Signal Specification : SignalSpecification  Unit=Pa
  Prs : Outport
  ScaleFctrs : Outport  Port=2
  wires:
  Signal Specification/1 -> Prs/1
  Gain/1 -> ScaleFctrs/1
  Front Pressure/1 -> Signal Specification/1
  Add/1 -> Gain/1
  lamda_mu_x/1 -> Add/1
  lamda_mu_y/1 -> Add/2

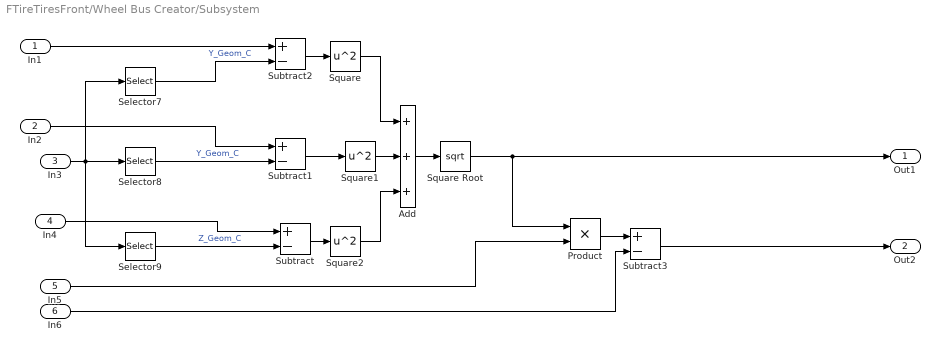
== system FTireTiresFront/Wheel Bus Creator/Subsystem ==
  In1 : Inport
  In2 : Inport  Port=2
  In3 : Inport  Port=3
  In4 : Inport  Port=4
  In5 : Inport  Port=5
  In6 : Inport  Port=6
  Add : Sum  Inputs=+++
  Product : Product
  Selector7 : Selector  NumberOfDimensions=2  IndexOptions=Index vector (dialog),Select all  Indices=26,1  OutputSizes=1,1
  Selector8 : Selector  NumberOfDimensions=2  IndexOptions=Index vector (dialog),Select all  Indices=27,1  OutputSizes=1,1
  Selector9 : Selector  NumberOfDimensions=2  IndexOptions=Index vector (dialog),Select all  Indices=28,1  OutputSizes=1,1
  Square : Math  Operator=square
  Square Root : Sqrt
  Square1 : Math  Operator=square
  Square2 : Math  Operator=square
  Subtract{,1..3} (4 alike) : Sum  Inputs=+-
  Out1 : Outport
  Out2 : Outport  Port=2
  wires:
  Selector9/1 -> Subtract/2  "Z_Geom_C"
  In3/1 -> Selector8/1, Selector9/1, Selector7/1
  Add/1 -> Square Root/1
  Square2/1 -> Add/3
  Selector7/1 -> Subtract2/2  "Y_Geom_C"
  In2/1 -> Subtract1/1
  Product/1 -> Subtract3/1
  Subtract1/1 -> Square1/1
  Subtract/1 -> Square2/1
  Selector8/1 -> Subtract1/2  "Y_Geom_C"
  Subtract2/1 -> Square/1
  Square/1 -> Add/1
  Square1/1 -> Add/2
  Square Root/1 -> Out1/1, Product/1
  In1/1 -> Subtract2/1
  In4/1 -> Subtract/1
  In5/1 -> Product/2
  Subtract3/1 -> Out2/1
  In6/1 -> Subtract3/2
